simulink model "Avi_DynamicBraking"  (Simulink 7.3)
settings: Solver=ode23tb  StartTime=0.0  StopTime=.03  RelTol=1e-3
libraries: powerlib x14
settings Model: Creator=Infosys  LastModifiedBy=Infosys

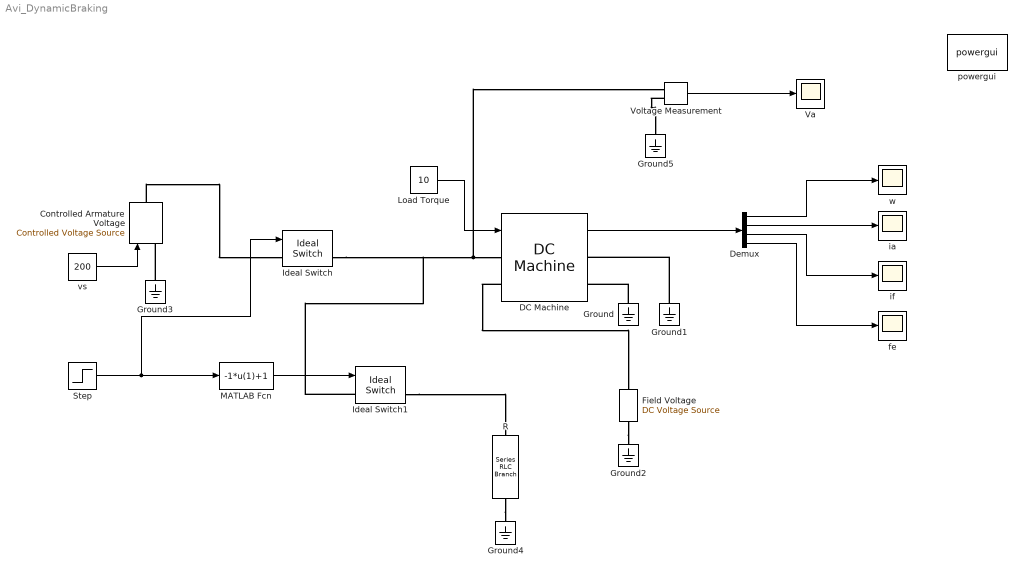
== system Avi_DynamicBraking ==
  Controlled Armature Voltage : powerlib/Electrical Sources/Controlled Voltage Source  DialogController=POWERSYS.PowerSysDialog  SystemSampleTime=-1  Initialize=on  Source_Type=DC  Amplitude=1  Phase=0  Frequency=0  Measurements=None
  DC Machine : powerlib/Machines/DC Machine  DialogController=POWERSYS.PowerSysDialog  SystemSampleTime=-1  PresetModel=02: 5HP 240V 1750RPM Field:150V  MechanicalLoad=Torque TL  ShowDetailedParameters=on  RLa=[0.78 0.016]  RLf=[150 112.5]  Laf=1.234  J=0.05  Bm=0.01  Tf=0  w0=0  Ifinit=1.33333333333333  TsPowergui=0  TsBlock=-1
  Demux : Demux
  Field Voltage : powerlib/Electrical Sources/DC Voltage Source  DialogController=POWERSYS.PowerSysDialog  SystemSampleTime=-1  Amplitude=200  Measurements=None
  Ground{,1..5} (6 alike) : powerlib/Elements/Ground  DialogController=POWERSYS.PowerSysDialog  PhysicalDomain=powersysdomain  SubClassName=unknown  LeftPortType=p1  RightPortType=p1  LConnTagsString=a
  Ideal Switch : powerlib/Power Electronics/Ideal Switch  DialogController=POWERSYS.PowerSysDialog  SystemSampleTime=-1  Ron=0.01  Lon=0  IC=0  Rs=.1  Cs=0.01e-6  Measurements=on
  Ideal Switch1 : powerlib/Power Electronics/Ideal Switch  DialogController=POWERSYS.PowerSysDialog  SystemSampleTime=-1  Ron=0.01  Lon=0  IC=0  Rs=.1  Cs=0.01e-6  Measurements=on
  Load Torque : Constant  Value=10  OutDataType=fixdt(1, 16)  OutScaling=2^0
  MATLAB Fcn : MATLABFcn  MATLABFcn=-1*u(1)+1
  R : powerlib/Elements/Series RLC Branch  DialogController=POWERSYS.PowerSysDialog  PhysicalDomain=powersysdomain  SubClassName=unknown  LeftPortType=p1  RightPortType=p1  LConnTagsString=__new0  RConnTagsString=__new0  BranchType=R  Resistance=50  Inductance=1e-3  SetiL0=off  InitialCurrent=0  Capacitance=1e-6  Setx0=off  InitialVoltage=0  Measurements=None
  Step : Step  SampleTime=0
  Va : Scope
  Voltage Measurement : powerlib/Measurements/Voltage Measurement  DialogController=POWERSYS.PowerSysDialog  SystemSampleTime=-1  PhasorSimulation=off  OutputType=Complex  PSBequivalent=0
  fe : Scope
      settings: SaveName=ScopeData4
  ia : Scope
      settings: SaveName=ScopeData2
  if : Scope
      settings: SaveName=ScopeData3
  powergui : powerlib/powergui  Priority=1  SystemSampleTime=-1  SimulationMode=Continuous  SampleTime=50e-6  frequency=60  SPID=off  DisableSnubberDevices=off  DisableRonSwitches=off  DisableVfSwitches=off  SwTol=0  Interpol=off  frequencyindice=0  echomessages=off  HookPort=off  DisplayEquations=off  FunctionMessages=off  EnableUseOfTLC=off  x0status=blocks  RestoreLinks=warning  Frange=[0:2:500]  Ylog=off  Xlog=on  ShowGrid=off  save=off  variable=ZData  ZoomFFT=on  StartTime=0.0  cycles=1  DisplayStyle=1  fundamental=60  FreqAxis=off  MaxFrequency=1000  frequencyindicesteady=1  RmsSteady=1  display=off  Ts=0  methode=off
  vs : Constant  Value=200  OutDataType=fixdt(1, 16)  OutScaling=2^0
  w : Scope
  wires:
  Load Torque/1 -> DC Machine/1
  vs/1 -> Controlled Armature Voltage/1
  MATLAB Fcn/1 -> Ideal Switch1/1
  Step/1 -> MATLAB Fcn/1, Ideal Switch/1
  DC Machine/1 -> Demux/1
  Voltage Measurement/1 -> Va/1
  Demux/1 -> w/1
  Demux/2 -> ia/1
  Demux/3 -> if/1
  Demux/4 -> fe/1
  connections:
  Ground/LConn1 -- DC Machine/RConn2
  Ground1/LConn1 -- DC Machine/RConn1
  DC Machine/LConn2 -- Field Voltage/RConn1
  Field Voltage/LConn1 -- Ground2/LConn1
  Ideal Switch1/LConn1 -- Ideal Switch/RConn1 -- DC Machine/LConn1 -- Voltage Measurement/LConn1
  Controlled Armature Voltage/RConn1 -- Ideal Switch/LConn1
  Ground3/LConn1 -- Controlled Armature Voltage/LConn1
  Ideal Switch1/RConn1 -- R/LConn1
  R/RConn1 -- Ground4/LConn1
  Voltage Measurement/LConn2 -- Ground5/LConn1
